simulink subsystem "AdjustEnvDelayParam"  (R2024a)
settings: Solver=VariableStepAuto  StartTime=0.0  StopTime=10.0  RelTol=1e-3
undefined symbols (not defined in the file or in its folder): max_delay_sec, sampling_freq
settings Model: Creator=david  LastModifiedBy=david

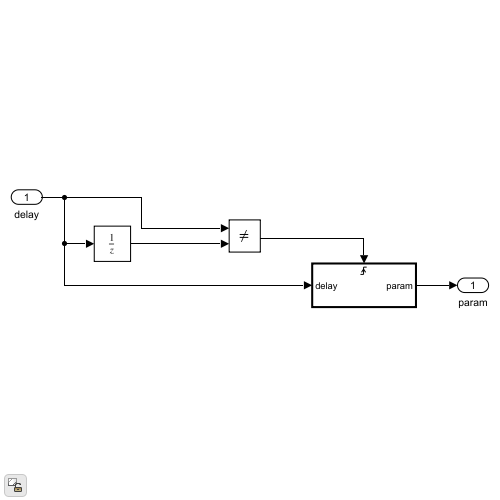
[thumbnail: Simulink's stored preview of the top-level diagram]
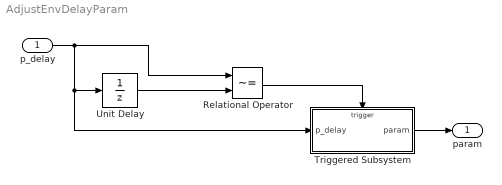
== system AdjustEnvDelayParam ==
  p_delay : Inport
  Relational Operator : RelationalOperator  Operator=~=  OutDataTypeStr=boolean  RndMeth=Simplest  InputSameDT=off
  Triggered Subsystem : Subsystem  TreatAsAtomicUnit=on
  Unit Delay : UnitDelay  SampleTime=-1  HasFrameUpgradeWarning=on
  param : Outport
  wires:
  p_delay/1 -> Relational Operator/1, Unit Delay/1, Triggered Subsystem/1(p_delay)
  Unit Delay/1 -> Relational Operator/2
  Relational Operator/1 -> Triggered Subsystem/Trigger
  Triggered Subsystem/1(param) -> param/1

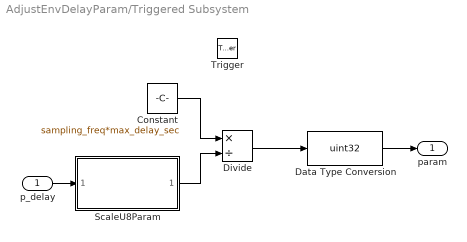
== system AdjustEnvDelayParam/Triggered Subsystem ==
  p_delay : Inport
  Trigger : TriggerPort  VariantControl=(inherit)  InitialTriggerSignalState=zero
  Constant : Constant  Value=sampling_freq*max_delay_sec  OutDataTypeStr=single
  Data Type Conversion : DataTypeConversion  OutDataTypeStr=uint32  SaturateOnIntegerOverflow=off  RndMeth=Floor
  Divide : Product  Inputs=*/
  ScaleU8Param : Subsystem  ReferencedSubsystem=ScaleU8Param
  param : Outport
  wires:
  Divide/1 -> Data Type Conversion/1
  ScaleU8Param/1 -> Divide/2
  p_delay/1 -> ScaleU8Param/1
  Constant/1 -> Divide/1
  Data Type Conversion/1 -> param/1
